simulink model "Khan_project_1_F4_model_v03"  (R2021a)
settings: Solver=ode4  StartTime=0.0  StopTime=t_final  FixedStep=t_step  RelTol=1e-3
undefined symbols (not defined in the file or in its folder): g, mass, q0, U1, VP_1, W1
libraries: sharedtransform x1
settings Model: Creator=ARK  LastModifiedBy=abdul
settings DataIOCC: ReturnWorkspaceOutputs=off

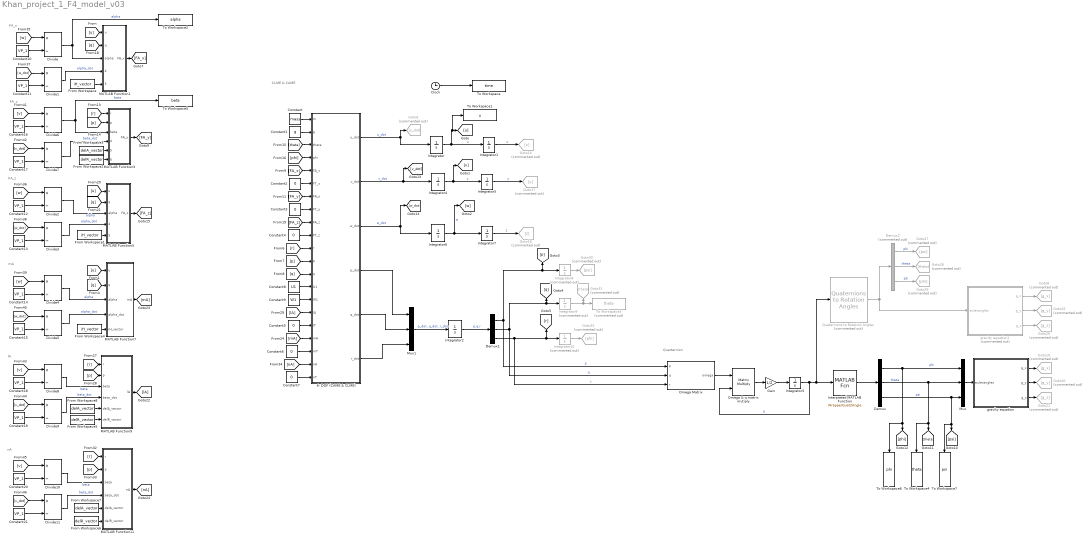
== system Khan_project_1_F4_model_v03 ==
  note: CLME & CAME
  note: nA
  note: lA
  note: mA
  note: Quarternion
  note: FA_z
  note: FA_y
  note: FA_x
  6- DOF (CAME & CLME) : MATLAB Function  TreatAsAtomicUnit=on
  Clock : Clock
  Constant : Constant  Value=mass
  Constant1 : Constant  Value=g
  Constant{10..21} (12 alike) : Constant  Value=VP_1
  Constant{2..7} (6 alike) : Constant  Value=0
  Constant8 : Constant  Value=U1
  Constant9 : Constant  Value=W1
  Demux : Demux  Outputs=3
  Demux1 : Demux  Outputs=3
  Demux2 : Demux  Commented=on  Outputs=3
  Divide{,1..11} (12 alike) : Product  Inputs=*/
  From Workspace : FromWorkspace  VariableName=iH_vector
  From Workspace1 : FromWorkspace  VariableName=iH_vector
  From Workspace2 : FromWorkspace  VariableName=delR_vector
  From Workspace3 : FromWorkspace  VariableName=delA_vector
  From Workspace4 : FromWorkspace  VariableName=iH_vector
  From Workspace5 : FromWorkspace  VariableName=delR_vector
  From Workspace6 : FromWorkspace  VariableName=delR_vector
  From Workspace7 : FromWorkspace  VariableName=delA_vector
  From Workspace8 : FromWorkspace  VariableName=delA_vector
  Gain : Gain  Gain=1/2
  Goto16 : Goto  Commented=on  GotoTag=x
  Goto17 : Goto  Commented=on  GotoTag=y
  Goto18 : Goto  Commented=on  GotoTag=z
  Goto19 : Goto  Commented=on  GotoTag=g_x
  Goto20 : Goto  Commented=on  GotoTag=g_y
  Goto21 : Goto  Commented=on  GotoTag=g_z
  Goto25 : Goto  Commented=on  GotoTag=g_y
  Goto26 : Goto  Commented=on  GotoTag=g_z
  Goto27 : Goto  Commented=on  GotoTag=psi
  Goto28 : Goto  Commented=on  GotoTag=theta
  Goto29 : Goto  Commented=on  GotoTag=phi
  Goto30 : Goto  Commented=on  GotoTag=psi
  Goto31 : Goto  Commented=on  GotoTag=theta
  Goto32 : Goto  Commented=on  GotoTag=phi
  Goto6 : Goto  Commented=on  GotoTag=u_dot
  Goto8 : Goto  Commented=on  GotoTag=g_x
  Integrator{,1..2,4..7} (7 alike) : Integrator
  Integrator10 : Integrator  Commented=on
  Integrator3 : Integrator  InitialCondition=q0
  Integrator8 : Integrator  Commented=on
  Integrator9 : Integrator  Commented=on
  Interpreted MATLAB Function : MATLABFcn  MATLABFcn=WrapperQuat2Angle
  MATLAB Function1 : MATLAB Function  TreatAsAtomicUnit=on
  MATLAB Function11 : MATLAB Function  TreatAsAtomicUnit=on
  MATLAB Function3 : MATLAB Function  TreatAsAtomicUnit=on
  MATLAB Function5 : MATLAB Function  TreatAsAtomicUnit=on
  MATLAB Function7 : MATLAB Function  TreatAsAtomicUnit=on
  MATLAB Function9 : MATLAB Function  TreatAsAtomicUnit=on
  Mux : Mux  Inputs=3
  Mux1 : Mux  Inputs=3
  Omega & q matrix mutiply : Product  Multiplication=Matrix(*)
  Omega Matrix : MATLAB Function  TreatAsAtomicUnit=on
  Quaternions to Rotation Angles : sharedtransform/Quaternions to Rotation Angles  Commented=on  rotationOrder=ZYX  aMode=aMode
      settings: SourceProductBaseCode=AE,PW,DR,MT,UV,VE
  To Workspace : ToWorkspace  VariableName=time  SampleTime=-1
  To Workspace1 : ToWorkspace  VariableName=u  SampleTime=-1
  To Workspace2 : ToWorkspace  VariableName=alpha  SampleTime=-1
  To Workspace3 : ToWorkspace  Commented=on  VariableName=theta  SampleTime=-1
  To Workspace4 : ToWorkspace  VariableName=theta  SampleTime=-1
  To Workspace5 : ToWorkspace  VariableName=beta  SampleTime=-1
  To Workspace6 : ToWorkspace  VariableName=phi  SampleTime=-1
  To Workspace7 : ToWorkspace  VariableName=psi  SampleTime=-1
  gravity equation : MATLAB Function  TreatAsAtomicUnit=on
  gravity equation1 : MATLAB Function  Commented=on  TreatAsAtomicUnit=on
  wires:
  6- DOF (CAME & CLME)/2(v_dot) -> [v_dot], Integrator4/1  "v_dot"
  6- DOF (CAME & CLME)/1(u_dot) -> Integrator/1, Goto6/1  "u_dot"
  Integrator/1 -> Integrator1/1, To Workspace1/1, [u]  "u"
  Integrator1/1 -> Goto16/1  "x"
  6- DOF (CAME & CLME)/4(p_dot) -> Mux1/1
  6- DOF (CAME & CLME)/5(q_dot) -> Mux1/2
  6- DOF (CAME & CLME)/6(r_dot) -> Mux1/3
  Mux1/1 -> Integrator2/1  "p_dot, q_dot, r_dot"
  Integrator2/1 -> Demux1/1  "p,q,r"
  Demux1/1 -> Integrator8/1, [p], Omega Matrix/1(p)  "p"
  Demux1/3 -> [r], Integrator10/1, Omega Matrix/3(r)  "r"
  Demux1/2 -> [q], Integrator9/1, Omega Matrix/2(q)  "q"
  Omega Matrix/1(omega) -> Omega & q matrix mutiply/1
  Omega & q matrix mutiply/1 -> Gain/1
  Gain/1 -> Integrator3/1
  Integrator3/1 -> Quaternions to Rotation Angles/1, Interpreted MATLAB Function/1, Omega & q matrix mutiply/2  "q"
  gravity equation/1(g_x) -> Goto19/1
  gravity equation/2(g_y) -> Goto20/1
  gravity equation/3(g_z) -> Goto21/1
  Constant/1 -> 6- DOF (CAME & CLME)/1(m)
  Integrator5/1 -> Goto17/1  "y"
  Integrator4/1 -> [v], Integrator5/1  "v"
  6- DOF (CAME & CLME)/3(w_dot) -> Integrator6/1, [w_dot]  "w_dot"
  Integrator7/1 -> Goto18/1  "z"
  Integrator6/1 -> [w], Integrator7/1  "w"
  [u] -> MATLAB Function1/1(u)
  Clock/1 -> To Workspace/1
  Constant1/1 -> 6- DOF (CAME & CLME)/2(g)
  [r] -> 6- DOF (CAME & CLME)/11(r)
  [q] -> 6- DOF (CAME & CLME)/13(q)
  [p] -> 6- DOF (CAME & CLME)/12(p)
  MATLAB Function1/1(FA_x) -> [FA_x]
  [FA_x] -> 6- DOF (CAME & CLME)/5(FA_x)
  Constant2/1 -> 6- DOF (CAME & CLME)/6(FT_x)
  Constant3/1 -> 6- DOF (CAME & CLME)/8(FT_y)
  Constant4/1 -> 6- DOF (CAME & CLME)/10(FT_z)
  MATLAB Function3/1(FA_y) -> [FA_y]
  [FA_y] -> 6- DOF (CAME & CLME)/7(FA_y)
  [p] -> MATLAB Function3/2(p)
  [r] -> MATLAB Function3/1(r)
  Demux/2 -> Mux/2, To Workspace4/1, [theta]  "theta"
  Demux/1 -> Mux/1, To Workspace6/1, [phi]  "phi"
  Demux/3 -> Mux/3, To Workspace7/1, [psi]  "psi"
  Mux/1 -> gravity equation/1(eulerangles)
  [theta] -> 6- DOF (CAME & CLME)/3(theta)
  [phi] -> 6- DOF (CAME & CLME)/4(phi)
  [q] -> MATLAB Function1/2(q)
  [FA_z] -> 6- DOF (CAME & CLME)/9(FA_z)
  [u] -> MATLAB Function5/1(u)
  [q] -> MATLAB Function5/2(q)
  MATLAB Function5/1(FA_z) -> [FA_z]
  From Workspace/1 -> MATLAB Function1/5(iH_vector)
  From Workspace1/1 -> MATLAB Function5/5(iH_vector)
  Constant8/1 -> 6- DOF (CAME & CLME)/14(U1)
  Constant5/1 -> 6- DOF (CAME & CLME)/17(lT)
  Constant6/1 -> 6- DOF (CAME & CLME)/19(mT)
  Constant7/1 -> 6- DOF (CAME & CLME)/21(nT)
  [u] -> MATLAB Function7/1(u)
  [q] -> MATLAB Function7/2(q)
  From Workspace4/1 -> MATLAB Function7/5(iH_vector)
  MATLAB Function7/1(mA) -> [mA]
  [mA] -> 6- DOF (CAME & CLME)/18(mA)
  [r] -> MATLAB Function9/1(r)
  MATLAB Function9/1(lA) -> [lA]
  [lA] -> 6- DOF (CAME & CLME)/16(lA)
  [p] -> MATLAB Function9/2(p)
  [p] -> MATLAB Function11/2(p)
  [r] -> MATLAB Function11/1(r)
  MATLAB Function11/1(nA) -> [nA]
  [nA] -> 6- DOF (CAME & CLME)/20(nA)
  From Workspace5/1 -> MATLAB Function9/6(delR_vector)
  From Workspace6/1 -> MATLAB Function11/6(delR_vector)
  From Workspace7/1 -> MATLAB Function11/5(delA_vector)
  From Workspace8/1 -> MATLAB Function9/5(delA_vector)
  Constant9/1 -> 6- DOF (CAME & CLME)/15(W1)
  From Workspace2/1 -> MATLAB Function3/6(delR_vector)
  Quaternions to Rotation Angles/1 -> gravity equation1/1(eulerangles), Demux2/1
  gravity equation1/3(g_z) -> Goto26/1
  gravity equation1/2(g_y) -> Goto25/1
  gravity equation1/1(g_x) -> Goto8/1
  Demux2/2 -> Goto28/1  "theta"
  Demux2/1 -> Goto27/1  "phi"
  Demux2/3 -> Goto29/1  "psi"
  [w] -> Divide/1
  Constant10/1 -> Divide/2
  Divide/1 -> To Workspace2/1, MATLAB Function1/3(alpha)  "alpha"
  Constant11/1 -> Divide1/2
  [w_dot] -> Divide1/1
  Constant13/1 -> Divide3/2
  [w_dot] -> Divide3/1
  [w] -> Divide2/1
  Constant12/1 -> Divide2/2
  Constant15/1 -> Divide5/2
  [w_dot] -> Divide5/1
  [w] -> Divide4/1
  Constant14/1 -> Divide4/2
  From Workspace3/1 -> MATLAB Function3/5(delA_vector)
  Divide2/1 -> MATLAB Function5/3(alpha)  "alpha"
  Divide3/1 -> MATLAB Function5/4(alpha_dot)  "alpha_dot"
  Divide4/1 -> MATLAB Function7/3(alpha)  "alpha"
  Divide5/1 -> MATLAB Function7/4(alpha_dot)  "alpha_dot"
  [v_dot] -> Divide7/1
  Constant17/1 -> Divide7/2
  Constant16/1 -> Divide6/2
  [v] -> Divide6/1
  Divide6/1 -> To Workspace5/1, MATLAB Function3/3(beta)  "beta"
  Divide7/1 -> MATLAB Function3/4(beta_dot)  "beta_dot"
  [v_dot] -> Divide9/1
  Constant19/1 -> Divide9/2
  [v] -> Divide8/1
  Constant18/1 -> Divide8/2
  Divide8/1 -> MATLAB Function9/3(beta)  "beta"
  Divide9/1 -> MATLAB Function9/4(beta_dot)  "beta_dot"
  [v_dot] -> Divide11/1
  Constant21/1 -> Divide11/2
  [v] -> Divide10/1
  Constant20/1 -> Divide10/2
  Divide10/1 -> MATLAB Function11/3(beta)  "beta"
  Divide11/1 -> MATLAB Function11/4(beta_dot)  "beta_dot"
  Integrator8/1 -> Goto30/1
  Integrator9/1 -> To Workspace3/1, Goto31/1
  Integrator10/1 -> Goto32/1
  Interpreted MATLAB Function/1 -> Demux/1
  Divide1/1 -> MATLAB Function1/4(alpha_dot)  "alpha_dot"

== matlab function Khan_project_1_F4_model_v03/MATLAB Function3 ==
  data: r input; FA_y output; p input; beta input; beta_dot input; delA_vector input; delR_vector input
function FA_y = fcn(r,p,beta,beta_dot,delA_vector,delR_vector)

    q_bar = 283;
    S = 530;
    CY_Beta = -0.478910835205265;
    b = 38.7;
    VP_1 = 875.6; %constant from speed (mach). From altitude and mach online calculator
    CY_r = 0.273949852132023;
    CY_delta_A = 0;
    C_Y_delta_R = 0.079243207607638;
    CY_beta_dot = 0;


FA_y = q_bar*S*(CY_Beta*beta+CY_beta_dot*((beta_dot*b)/(2*VP_1))+CY_r*((p*b)/(2*VP_1))+ ...
    CY_r*((r*b)/(2*VP_1))+CY_delta_A*delA_vector+C_Y_delta_R*delR_vector);

== matlab function Khan_project_1_F4_model_v03/MATLAB Function5 ==
  data: u input; FA_z output; q input; alpha input; alpha_dot input; iH_vector input
function FA_z = fcn(u,q,alpha,alpha_dot,iH_vector)
    
    q_bar = 283;
    S = 530;
    VP_1 = 875.6;
    CL_alphadot = 0.918177277267356;
    c_bar = 16;
    CL_q = 3.604489646224828;
    CL_delta_E = 0;
    CL_u = 0;
    CL_1 = 0;
    CL_alpha = 0;
    CD_one = 0;
    delta_E = 0;
    CL_i_H = 0.528809892965624;
    

FA_z = q_bar*S*(-(CL_u + 2*CL_1)*(u/VP_1)+(-CL_alpha+CD_one)*alpha ...
    -CL_alphadot*((alpha_dot*c_bar)/(2*VP_1))-CL_q*((q*c_bar)/(2*VP_1))-CL_delta_E*delta_E-CL_i_H*iH_vector);

== matlab function Khan_project_1_F4_model_v03/MATLAB Function7 ==
  data: u input; q input; mA output; alpha input; alpha_dot input; iH_vector input
function mA = fcn(u,q,alpha,alpha_dot,iH_vector)

    q_bar =   283.2000;
    S = 530;
    VP_1 = 875.6000;
    c_bar = 16;
    Cm_q =    -1.8921;
    Cm_alpha =    -1.8921;
    Cm_alphadot = -1.092067765566989;
    Cm_iH = -0.656071535872698;
    Cm_delta_E = 0;
    delta_E = 0;
    xbar_AC_W = 0.363520000000000;
    CL_one = 0.2598;
    mach = 0.9;
    Cm_u = -CL_one*(xbar_AC_W/mach);
    Cm_1 = 0;


 mA = q_bar*S*c_bar*([Cm_u+2*Cm_1]*(u/VP_1)+Cm_alpha*alpha+Cm_alphadot*((alpha_dot*c_bar)/(2*VP_1))...
     +Cm_q*((q*c_bar)/(2*VP_1))+Cm_delta_E*delta_E + Cm_iH*iH_vector);

== matlab function Khan_project_1_F4_model_v03/MATLAB Function9 ==
  data: r input; lA output; p input; beta input; beta_dot input; delA_vector input; delR_vector input
function lA = fcn(r,p,beta,beta_dot,delA_vector,delR_vector)

    q_bar = 283;
    S = 530;
    b = 38.7;
    VP_1 = 875.6;
    CL_Beta = -0.153857650789122;
    CL_betadot = 0;
    CL_p =-0.167124467253975;
    CL_r = 0.173395603243981;
    CL_delta_A = 0.026100000000000;
    CL_delta_R = 0.012628913286059;

lA = q_bar*S*b*(CL_Beta*beta+CL_betadot*((beta_dot*b)/(2*VP_1))+CL_p*((p*b)/(2*VP_1)) ...
    + CL_r*((r*b)/(2*VP_1))+ CL_delta_A *delA_vector + CL_delta_R *delR_vector);

== matlab function Khan_project_1_F4_model_v03/MATLAB Function11 ==
  data: r input; nA output; p input; beta input; beta_dot input; delA_vector input; delR_vector input
function nA = fcn(r,p,beta,beta_dot,delA_vector,delR_vector)

    q_bar = 283;
    S = 530;
    b = 38.7;
    VP_1 = 875.6;
    Cn_Beta = 0.045700548741188;
    Cn_betadot = 0;
    Cn_p = -0.053979762256550;
    Cn_r = -0.101036057614036;
    Cn_delta_A = 6.759900000000001e-05;
    Cn_delta_R = -0.055916406077118;

nA = q_bar*S*b*(Cn_Beta*beta+Cn_betadot*((beta_dot*b)/(2*VP_1))+Cn_p*((p*b)/(2*VP_1)) ...
    + Cn_r*((r*b)/(2*VP_1))+ Cn_delta_A*delA_vector + Cn_delta_R*delR_vector);

== matlab function Khan_project_1_F4_model_v03/gravity equation1 ==
  data: eulerangles input; g_x output; g_y output; g_z output
function [g_x,g_y,g_z] = fcn(eulerangles)

    g = 9.81;
g_x = -g*sin(eulerangles(2));
g_y = g*cos(eulerangles(2))*sin(eulerangles(1));
g_z = g*cos(eulerangles(2))*cos(eulerangles(1));

== matlab function Khan_project_1_F4_model_v03/Omega Matrix ==
  data: p input; omega output; q input; r input
function omega = fcn(p,q,r)


wx = p;
wy = q;
wz = r;
omega = [0 -wx -wy -wz;
    wx 0 wz -wy;
    wy -wz 0 wx;
    wz wy -wx 0];

== matlab function Khan_project_1_F4_model_v03/6- DOF (CAME & CLME) ==
  data: m input; u_dot output; v_dot output; w_dot output; g input; theta input; phi input; FA_x input; FT_x input; FA_y input; FT_y input; FA_z input; FT_z input; r input; p input; q input; p_dot output; q_dot output; r_dot output; U1 input; W1 input; lA input; lT input; mA input; mT input; nA input; nT input



function [u_dot,v_dot,w_dot,p_dot,q_dot,r_dot] = fcn(m,g,theta,phi,FA_x,FT_x,FA_y,FT_y,FA_z,FT_z,r,p,q,U1,W1,lA,lT,mA,mT,nA,nT)

    VP_1 = 875.6; 
    alpha_1 = 0.045378560551853;
    theta_one = 0;
    Ixx = 23700;
    Ixz = 1600;
    Iyy = 117500;
    Izz = 133700;

    % CLMEs
    u_dot = (1/m)*(-m*g*theta*cos(theta_one)+(FA_x+FT_x))-(q*W1); %This is correct
%     u_dot = (-g*theta)+(FA_x/m)-(q*W1)
    v_dot = (1/m)*(m*g*phi*cos(theta_one)+(FA_y+FT_y))-(U1*r)+(p*W1);
    w_dot = (1/m)*(-m*g*theta*sin(theta_one)+(FA_z+FT_z))+(U1*q);

    %CAMEs
    % [We are doing CAMEs. So KEs,GEs, and FPEs]
    % p_dot = (1/Ixx)*((r_dot*Ixz)+(p*q*Ixz)-((r*q)*(I_ZZ-Iyy))+L_A+L_T);
    % q_dot = (1/Iyy)*((-p*r*(Ixx-Izz))-(Ixz*(p^2-r^2))+M_A+M_T);
    % r_dot = (1/Izz)*((p_dot*Ixz)-(p*q)*(Iyy-Ixx)-(q*r*Ixz)+N_A+N_T);

    A = [Ixx 0 -Ixz;0 Iyy 0; -Ixz 0 Izz];
    % x = [p_dot; q_dot; r_dot]; % we are solving for this section so it needs
    % to be commented out
    B = [lA + lT; mA + mT; nA + nT];

x = inv(A)*B;
p_dot = x(1);
q_dot = x(2);
r_dot = x(3);

== matlab function Khan_project_1_F4_model_v03/gravity equation ==
  data: eulerangles input; g_x output; g_y output; g_z output
function [g_x,g_y,g_z] = fcn(eulerangles)

g = 9.81;

g_x = -g*sin(eulerangles(2));
g_y = g*cos(eulerangles(2))*sin(eulerangles(1));
g_z = g*cos(eulerangles(2))*cos(eulerangles(1));

== matlab function Khan_project_1_F4_model_v03/MATLAB Function1 ==
  data: u input; q input; FA_x output; alpha input; alpha_dot input; iH_vector input
function FA_x = fcn(u,q,alpha,alpha_dot,iH_vector)

    q_bar = 283;
    weight = 39000;
    S = 530;
    CD_alpha = 0.226818363884153;
    c_bar = 16;
    delta_E = 0;
    CD_u = 0;
    Cd_1 = 0;
    VP_1 = 875.6; %constant from speed (mach). From altitude and mach online calculator
    CL_one = weight/(q_bar*S);
    CD_q = 0;% zero from book
    CD_delta_E = 0;% zero from book
    CD_i_H = -0.1; % Ask if it is negative or not
    
    
FA_x = q_bar*S*(-(CD_u + 2*Cd_1)*(u/VP_1)+(-CD_alpha+CL_one)*alpha ...
    -CD_alpha*((alpha_dot*c_bar)/(2*VP_1))-CD_q*((q*c_bar)/(2*VP_1))-CD_delta_E*delta_E-CD_i_H*iH_vector);
